simulink model "usv_sys"  (R2023b)
settings: Solver=VariableStepAuto  StartTime=0.0  StopTime=200  RelTol=1e-3
libraries: slpidlib x1
settings Model: Creator=hw  LastModifiedBy=hw

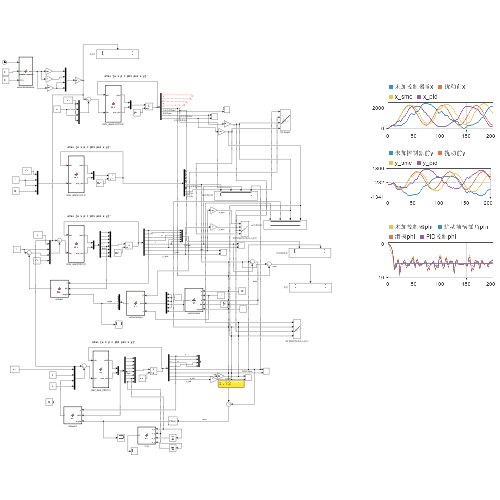
[thumbnail: Simulink's stored preview of the top-level diagram]
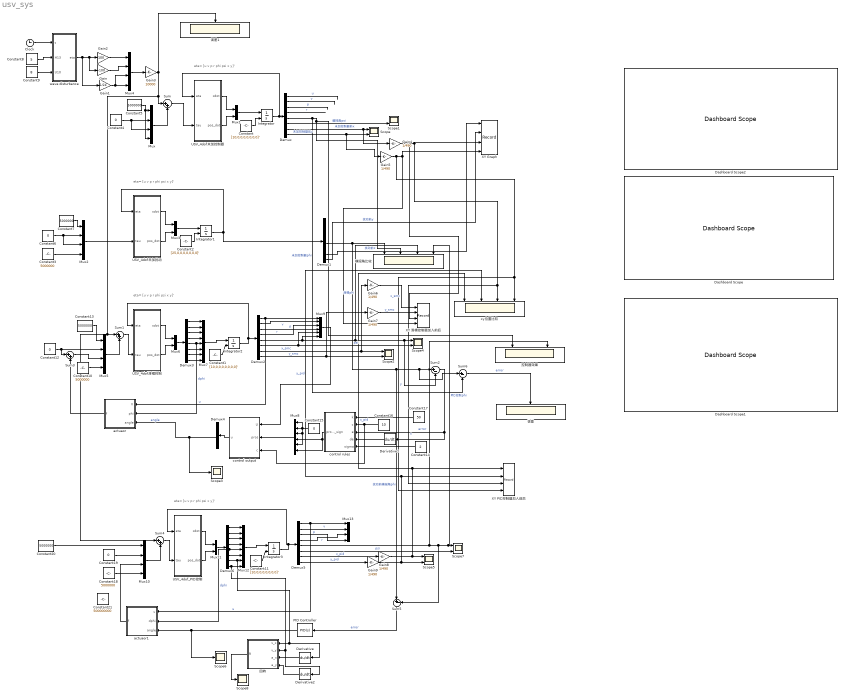
== system usv_sys ==
  note: eta= [u v p r phi psi x y]'
  note: eta= [u v p r phi psi x y]'
  note: eta= [u v p r phi psi x y]'
  note: eta= [u v p r phi psi x y]'
  Clock : Clock
  Constant : Constant  Value=[10,0,0,0,0,0,0,0]'  VectorParams1D=off
  Constant1 : Constant  Value=[10,0,0,0,0,0,0,0]'  VectorParams1D=off
  Constant{3,5,7,10,13,18,20} (7 alike) : Constant  Value=5000000
  Constant11 : Constant  Value=[10,0,0,0,0,0,0,0]'  VectorParams1D=off
  Constant{4,6,12,15,19} (5 alike) : Constant  Value=0
  Constant14 : Constant  Value=2
  Constant16 : Constant  Value=10
  Constant17 : Constant  Value=50
  Constant2 : Constant  Value=[25,0,0,0,0,0,0,0]'  VectorParams1D=off
  Constant21 : Constant  Value=500000000
  Constant8 : Constant  Value=5
  Constant9 : Constant  Value=8
  Dashboard Scope : DashboardScope
  Dashboard Scope1 : DashboardScope
  Dashboard Scope2 : DashboardScope
  Demux{,1..3,5..6} (6 alike) : Demux  Outputs=8
  Demux4 : Demux  Outputs=6
  Derivative : Derivative
  Derivative1 : Derivative
  Derivative2 : Derivative
  Gain : Gain  Gain=-100
  Gain1 : Gain  Gain=1/24
  Gain2 : Gain  Gain=100
  Gain3 : Gain  Gain=10000
  Gain{4..9} (6 alike) : Gain  Gain=1/490
  Integrator{,1..3} (4 alike) : Integrator  InitialConditionSource=external
  Mux{,2,4..5,10,13} (6 alike) : Mux
  Mux{1,3,6,11} (4 alike) : Mux  Inputs=2
  Mux12 : Mux  Inputs=8
  Mux7 : Mux  Inputs=8
  Mux8 : Mux  Inputs=6
  Mux9 : Mux  Inputs=6
  PID Controller : slpidlib/PID Controller  Controller=PID  Form=Parallel  TimeDomain=Continuous-time  UseExternalTs=off  SampleTime=-1  IntegratorMethod=Forward Euler  FilterMethod=Forward Euler  ControllerParametersSource=internal  P=5  I=0.01  UseKiTs=off  D=2  N=100  UseFilter=on  TunerSelectOption=Transfer Function Based (PID Tuner App)  InitialConditionSource=internal  InitialConditionForIntegrator=0  InitialConditionForFilter=0  DifferentiatorICPrevScaledInput=0  ExternalReset=none  TrackingMode=off  Kt=1  LimitOutput=off  SatLimitsSource=internal  UpperSaturationLimit=inf  LowerSaturationLimit=-inf  LinearizeAsGain=on  AntiWindupMode=none  Kb=1  LimitIntegrator=off  UpperIntegratorSaturationLimit=inf  LowerIntegratorSaturationLimit=-inf  POutMin=[]  POutMax=[]  IOutMin=[]  IOutMax=[]  DOutMin=[]  DOutMax=[]  NOutMin=[]  NOutMax=[]  SumOutMin=[-15]  SumOutMax=[15]  SaturationOutMin=[]  SaturationOutMax=[]  PParamMin=[]  PParamMax=[]  IParamMin=[]  IParamMax=[]  DParamMin=[]  DParamMax=[]  NParamMin=[]  NParamMax=[]  KbParamMin=[]  KbParamMax=[]  KtParamMin=[]  KtParamMax=[]  KbOutMin=[]  KbOutMax=[]  KtOutMin=[]  KtOutMax=[]  IntegratorOutMin=[]  IntegratorOutMax=[]  FilterOutMin=[]  FilterOutMax=[]  SumI1OutMin=[]  SumI1OutMax=[]  SumI2OutMin=[]  SumI2OutMax=[]  SumI3OutMin=[]  SumI3OutMax=[]  SumI4OutMin=[]  SumI4OutMax=[]  SumDOutMin=[]  SumDOutMax=[]  DifferentiatorOutMin=[]  DifferentiatorOutMax=[]  FilterDiffOutCoefMin=[]  FilterDiffOutCoefMax=[]  ReciprocalOutMin=[]  ReciprocalOutMax=[]  SumDenOutMin=[]  SumDenOutMax=[]  SumNumOutMin=[]  SumNumOutMax=[]  DivideOutMin=[]  DivideOutMax=[]  UdiffTsProdOutMin=[]  UdiffTsProdOutMax=[]  NTsProdOutMin=[]  NTsProdOutMax=[]  UintegralTsProdOutMin=[]  UintegralTsProdOutMax=[]  UngainTsProdOutMin=[]  UngainTsProdOutMax=[]  ClampingZeroOutDataTypeStr=Inherit: Inherit via back propagation  ClampingZeroOutMin=[]  ClampingZeroOutMax=[]  FilterDenConstantOutDataTypeStr=Inherit: Inherit via back propagation  FilterDenConstantOutMin=[]  FilterDenConstantOutMax=[]  PCopyOutDataTypeStr=Inherit: Inherit via back propagation  PCopyOutMin=[]  PCopyOutMax=[]  NCopyOutDataTypeStr=Inherit: Inherit via back propagation  NCopyOutMin=[]  NCopyOutMax=[]  IntegratorContinuousStateAttributes=''  IntegratorStateMustResolveToSignalObject=off  IntegratorRTWStateStorageClass=Auto  FilterContinuousStateAttributes=''  FilterStateMustResolveToSignalObject=off  FilterRTWStateStorageClass=Auto  ParallelPVariant=InternalParameters  IdealPVariant=Disabled  IVariant=InternalParameters  DVariant=InternalParameters  IntegratorVariant=Continuous  SatVariant=Disabled  AWVariant=Passthrough  PCopyVariant=Disabled  TRVariant=Disabled  FdbkBlocksVariant=Forward  IdealPFdbkVariant=Disabled  SatFdbkVariant=Disabled  DerivativeFilterVariant=ContFilter  NVariant=InternalParameters  NCopyVariant=Disabled  FilterICVariant=InternalICsFilter  IntegratorICVariant=InternalICs  ExternalResetVariant=Disabled  TRSumVariant=Passthrough  SumFdbkVariant=Disabled  SumVariant=Sum_PID  TsampFilterVariant=InternalTs  TsampNgainVariant=Passthrough  TsampIntegralVariant=Disabled_SignalSpec  ExternalSaturationOutDataTypeStr=Inherit: Same as second input
  Scope{,1..2,4..5,7} (6 alike) : Scope  NumInputPorts=2
  Scope3 : Scope
  Scope6 : Scope
  Scope8 : Scope
  Sum{,1,3..4} (4 alike) : Sum  Inputs=|++
  Sum2 : Sum  Inputs=|+-
  Sum5 : Sum  Inputs=|+-
  Sum6 : Sum  Inputs=|+-
  USV_4dof_PID控制 : MATLAB Function  TreatAsAtomicUnit=on
  USV_4dof未加扰动 : MATLAB Function  TreatAsAtomicUnit=on
  USV_4dof未加控制器 : MATLAB Function  TreatAsAtomicUnit=on
  USV_4dof滑模控制 : MATLAB Function  TreatAsAtomicUnit=on
  XY Graph : Record  RecordToFile=on  FileSettingsInternal="{\"entries\":[{\"content\":{\"excelSettings\":{\"content\":{},\"type\":\"Streamout.ExcelSettings\"}},\"type\":\"Streamout.FileSettingStorage\",\"uuid\":\"\"}],\"packageUris\":[\"http:\\/\\/schema.mathworks.com\\/mf0\\/streamout_blocks\\/R2020a\"],\"version\":\"1.0\"}"  Layout=[1 1]  SignalsInternal="{\"entries\":[{\"content\":{\"signals\":[{\"content\":{\"blockPath\":[],\"dimensions\":[1,1],\"domain\":\"\",\"lineColor\":\"#ff6929\",\"plots\":[1],\"port\":1,\"sid\":[\"\"],\"signalID\":6587,\"signalName\":\"扰动前x\"},\"type\":\"RecordBlkView.Signal\",\"uuid\":\"\"},{\"content\":{\"blockPath\":[],\"dimensions\":[1,1],\"domain\":\"\",\"lineColor\":\"#b746ff\",\"plots\":[1],\"port\":2,\"sid\":[\"\"],\"signalID\":6591,\"signalName\":\"扰动前y\"},\"type\":\"RecordBlkView.Signal\",\"uuid\":\"\"},{\"content\":{\"blockPath\":[],\"dimensions\":[1,1],\"domain\":\"\",\"lineColor\":\"#edb120\",\"port\":3,\"sid\":[\"\"],\"signalID\":6595,\"signalName\":\"x\"},\"type\":\"RecordBlkView.Signal\",\"uuid\":\"\"},{\"content\":{\"blockPath\":[],\"dimensions\":[1,1],\"domain\":\"\",\"lineColor\":\"#7e2f8e\",\"port\":4,\"sid\":[\"\"],\"signalID\":6599,\"signalName\":\"y\"},\"type\":\"RecordBlkView.Signal\",\"uuid\":\"\"}]},\"type\":\"RecordBlkView.InputSignals\",\"uuid\":\"\"}],\"packageUris\":[\"http:\\/\\/schema.mathworks.com\\/mf0\\/streamout_blocks\\/R2020a\"],\"version\":\"1.0\"}"  VisualizationBindings="{\"xyplotplugin\":{\"info\":[{\"series\":[{\"bindingParametersList\":[{\"parameter\":\"X-Axis\",\"signalID\":6587,\"signalName\":\"扰动前x\"},{\"parameter\":\"Y-Axis\",\"signalID\":6591,\"signalName\":\"扰动前y\"}],\"seriesID\":62716}],\"subplotID\":1}]}}"  CompatibilityTag=XY
  XY PID控制器加入前后 : Record  FileSettingsInternal="{\"entries\":[{\"content\":{\"excelSettings\":{\"content\":{},\"type\":\"Streamout.ExcelSettings\"}},\"type\":\"Streamout.FileSettingStorage\",\"uuid\":\"\"}],\"packageUris\":[\"http:\\/\\/schema.mathworks.com\\/mf0\\/streamout_blocks\\/R2020a\"],\"version\":\"1.0\"}"  Layout=[1 1]  SignalsInternal="{\"entries\":[{\"content\":{\"signals\":[{\"content\":{\"blockPath\":[],\"dimensions\":[1,1],\"domain\":\"\",\"lineColor\":\"#77ac30\",\"port\":1,\"sid\":[\"\"],\"signalID\":6603,\"signalName\":\"x_pid\"},\"type\":\"RecordBlkView.Signal\",\"uuid\":\"\"},{\"content\":{\"blockPath\":[],\"dimensions\":[1,1],\"domain\":\"\",\"lineColor\":\"#4dbeee\",\"port\":2,\"sid\":[\"\"],\"signalID\":6607,\"signalName\":\"y_pid\"},\"type\":\"RecordBlkView.Signal\",\"uuid\":\"\"},{\"content\":{\"blockPath\":[],\"dimensions\":[1,1],\"domain\":\"\",\"lineColor\":\"#a2142f\",\"port\":3,\"sid\":[\"\"],\"signalID\":6611,\"signalName\":\"x\"},\"type\":\"RecordBlkView.Signal\",\"uuid\":\"\"},{\"content\":{\"blockPath\":[],\"dimensions\":[1,1],\"domain\":\"\",\"lineColor\":\"#139fff\",\"port\":4,\"sid\":[\"\"],\"signalID\":6615,\"signalName\":\"y\"},\"type\":\"RecordBlkView.Signal\",\"uuid\":\"\"}]},\"type\":\"RecordBlkView.InputSignals\",\"uuid\":\"\"}],\"packageUris\":[\"http:\\/\\/schema.mathworks.com\\/mf0\\/streamout_blocks\\/R2020a\"],\"version\":\"1.0\"}"  VisualizationBindings="{\"xyplotplugin\":{\"info\":[{\"series\":[],\"subplotID\":1}]}}"  CompatibilityTag=XY
  XY 滑模控制器加入前后 : Record  FileSettingsInternal="{\"entries\":[{\"content\":{\"excelSettings\":{\"content\":{},\"type\":\"Streamout.ExcelSettings\"}},\"type\":\"Streamout.FileSettingStorage\",\"uuid\":\"\"}],\"packageUris\":[\"http:\\/\\/schema.mathworks.com\\/mf0\\/streamout_blocks\\/R2020a\"],\"version\":\"1.0\"}"  Layout=[1 1]  SignalsInternal="{\"entries\":[{\"content\":{\"signals\":[{\"content\":{\"blockPath\":[],\"dimensions\":[1,1],\"domain\":\"\",\"lineColor\":\"#4dbeee\",\"port\":1,\"sid\":[\"\"],\"signalID\":6619,\"signalName\":\"x_smc\"},\"type\":\"RecordBlkView.Signal\",\"uuid\":\"\"},{\"content\":{\"blockPath\":[],\"dimensions\":[1,1],\"domain\":\"\",\"lineColor\":\"#a2142f\",\"port\":2,\"sid\":[\"\"],\"signalID\":6623,\"signalName\":\"y_smc\"},\"type\":\"RecordBlkView.Signal\",\"uuid\":\"\"},{\"content\":{\"blockPath\":[],\"dimensions\":[1,1],\"domain\":\"\",\"lineColor\":\"#139fff\",\"port\":3,\"sid\":[\"\"],\"signalID\":6627,\"signalName\":\"x\"},\"type\":\"RecordBlkView.Signal\",\"uuid\":\"\"},{\"content\":{\"blockPath\":[],\"dimensions\":[1,1],\"domain\":\"\",\"lineColor\":\"#ff6929\",\"port\":4,\"sid\":[\"\"],\"signalID\":6631,\"signalName\":\"y\"},\"type\":\"RecordBlkView.Signal\",\"uuid\":\"\"}]},\"type\":\"RecordBlkView.InputSignals\",\"uuid\":\"\"}],\"packageUris\":[\"http:\\/\\/schema.mathworks.com\\/mf0\\/streamout_blocks\\/R2020a\"],\"version\":\"1.0\"}"  VisualizationBindings="{\"xyplotplugin\":{\"info\":[{\"series\":[],\"subplotID\":1}]}}"  CompatibilityTag=XY
  actuaor : MATLAB Function  TreatAsAtomicUnit=on
  actuaor1 : MATLAB Function  TreatAsAtomicUnit=on
  control output : MATLAB Function  TreatAsAtomicUnit=on
  control rules : MATLAB Function  TreatAsAtomicUnit=on
  wave disturbance : MATLAB Function  TreatAsAtomicUnit=on
  xy位置比较 : Scope  NumInputPorts=4
  回转 : MATLAB Function  TreatAsAtomicUnit=on
  控制器效果 : Scope  NumInputPorts=2
  横摇角比较 : Scope  NumInputPorts=4
  误差 : Scope
  误差1 : Scope
  wires:
  Constant/1 -> Integrator/2
  Constant4/1 -> Mux/3, Mux/2
  USV_4dof未加控制器/1(xdot) -> Mux1/1
  Demux/7 -> Gain4/1, Scope/1  "未加控制器前x"
  Demux/8 -> Gain5/1, Scope/2  "未加控制器前y"
  USV_4dof未加控制器/2(pos_dot) -> Mux1/2
  Constant5/1 -> Mux/4, Mux/1
  Integrator/1 -> USV_4dof未加控制器/1(eta), Demux/1
  Mux/1 -> Sum/2
  Mux1/1 -> Integrator/1
  Demux/1 -> ?  "u"
  Demux/2 -> ?  "v"
  Demux/3 -> ?  "p"
  Demux/4 -> ?  "r"
  Demux/6 -> Scope1/2  "艏摇角psi"
  Mux2/1 -> USV_4dof未加扰动/2(tau)
  USV_4dof未加扰动/2(pos_dot) -> Mux3/2
  Constant3/1 -> Mux2/4
  Constant7/1 -> Mux2/1
  USV_4dof未加扰动/1(xdot) -> Mux3/1
  Constant2/1 -> Integrator1/2
  Integrator1/1 -> USV_4dof未加扰动/1(eta), Demux1/1
  Constant6/1 -> Mux2/3, Mux2/2
  Mux3/1 -> Integrator1/1
  Constant9/1 -> wave disturbance/3(U10)
  Mux4/1 -> Gain3/1
  Gain1/1 -> Mux4/3, Mux4/4
  Clock/1 -> wave disturbance/1(t)
  Gain2/1 -> Mux4/1
  Constant8/1 -> wave disturbance/2(H13)
  wave disturbance/1(eta) -> Gain1/1, Gain/1, Gain2/1
  Sum/1 -> USV_4dof未加控制器/2(tau)
  Gain4/1 -> XY 滑模控制器加入前后/3, XY PID控制器加入前后/3, xy位置比较/3, XY Graph/3  "x"
  Gain5/1 -> XY PID控制器加入前后/4, xy位置比较/4, XY 滑模控制器加入前后/4, XY Graph/4  "y"
  Demux/5 -> Sum6/2, 控制器效果/1, 横摇角比较/2  "未加控制器phi"
  Demux1/5 -> Sum5/1, Sum6/1, Sum2/1, 横摇角比较/1  "扰动前横摇角phi"
  Demux2/6 -> Mux9/5, Scope4/2  "psi"
  Demux2/7 -> Scope2/1, Gain6/1  "x_smc"
  USV_4dof滑模控制/2(pos_dot) -> Mux6/2
  Demux2/4 -> Mux9/3  "r"
  Demux4/4 -> Scope3/1, actuaor/3(angle)  "angle"
  Constant13/1 -> Mux5/1
  Derivative1/1 -> control rules/4(de)
  Mux7/1 -> Integrator2/1
  Mux8/1 -> control output/2(pros)
  Demux3/7 -> Mux7/7
  Mux9/1 -> control output/1(U)
  Demux3/3 -> Mux7/3
  Demux2/2 -> Mux9/2  "v"
  Demux3/5 -> actuaor/2(phi), Mux7/5  "dphi"
  Constant17/1 -> control rules/1(k)
  Constant12/1 -> Sum3/1, Mux5/2
  Constant14/1 -> control rules/5(sigma)
  Demux2/1 -> actuaor/1(V), Mux9/1  "u"
  control rules/1(prox1_sign) -> Mux8/6, Mux8/4
  Sum2/1 -> Derivative1/1, control rules/3(e)  "error"
  Demux2/8 -> Gain7/1, Scope2/2  "y_smc"
  Constant1/1 -> Integrator2/2
  Sum3/1 -> Mux5/3
  Demux2/5 -> Mux9/6, Sum2/2, Scope4/1, 横摇角比较/3  "滑模phi"
  Demux3/6 -> Mux7/6
  Demux3/4 -> Mux7/4
  Demux2/3 -> Mux9/4  "p"
  Demux3/1 -> Mux7/1
  Constant15/1 -> Mux8/1, Mux8/5, Mux8/3, Mux8/2
  Demux3/2 -> Mux7/2
  Mux6/1 -> Demux3/1
  Constant16/1 -> control output/3(c), control rules/2(c)
  Constant10/1 -> Mux5/4
  Integrator2/1 -> USV_4dof滑模控制/1(eta), Demux2/1
  Demux3/8 -> Mux7/8
  actuaor/1(f) -> Sum3/2
  USV_4dof滑模控制/1(xdot) -> Mux6/1
  Mux5/1 -> Sum1/2
  Sum1/1 -> USV_4dof滑模控制/2(tau)
  control output/1(u) -> Demux4/1
  actuaor1/1(f) -> Mux10/3
  Gain3/1 -> Sum4/1, Sum1/1, Sum/1, 误差1/1
  回转/1(R) -> Scope8/1
  Integrator3/1 -> USV_4dof_PID控制/1(eta), Demux5/1
  Constant11/1 -> Integrator3/2
  USV_4dof_PID控制/2(pos_dot) -> Mux11/2
  Demux6/7 -> 回转/1(v_x), Derivative/1, Mux12/7
  Demux6/5 -> Mux12/5, actuaor1/2(dphi)  "dphi"
  Mux11/1 -> Demux6/1
  Demux6/2 -> Mux12/2
  Mux12/1 -> Integrator3/1
  PID Controller/1 -> Scope6/1, actuaor1/3(angle)
  Demux6/4 -> Mux12/4
  Demux5/5 -> 控制器效果/2, 横摇角比较/4, Scope7/1, Sum5/2  "PID控制phi"
  Constant18/1 -> Mux10/4
  Demux6/3 -> Mux12/3
  Demux5/8 -> Gain9/1  "y_pid"
  Demux5/1 -> Mux13/1, actuaor1/1(v)  "u"
  Demux5/4 -> Mux13/3  "r"
  Demux5/6 -> Scope7/2  "psi"
  Demux6/8 -> Derivative2/1, 回转/2(v_y), Mux12/8
  Demux5/2 -> Mux13/2  "v"
  Demux5/7 -> Gain8/1  "x_pid"
  Mux10/1 -> Sum4/2
  Constant20/1 -> Mux10/1
  Sum5/1 -> PID Controller/1  "error"
  Demux6/6 -> Mux12/6
  Derivative/1 -> 回转/3(a_x)
  Sum4/1 -> USV_4dof_PID控制/2(tau)
  USV_4dof_PID控制/1(xdot) -> Mux11/1
  Demux6/1 -> Mux12/1
  Constant19/1 -> Mux10/2
  Demux5/3 -> Mux13/4  "p"
  Derivative2/1 -> 回转/4(a_y)
  Gain/1 -> Mux4/2
  Gain6/1 -> XY 滑模控制器加入前后/1  "x_smc"
  Gain7/1 -> XY 滑模控制器加入前后/2  "y_smc"
  Gain8/1 -> XY PID控制器加入前后/1, xy位置比较/1, Scope5/1  "x_pid"
  Gain9/1 -> XY PID控制器加入前后/2, xy位置比较/2, Scope5/2  "y_pid"
  Sum6/1 -> 误差/1  "error"
  Demux1/7 -> XY Graph/1  "扰动前x"
  Demux1/8 -> XY Graph/2  "扰动前y"

== matlab function usv_sys/USV_4dof未加控制器 ==
  data: eta input size=8*1; xdot output size=6*1; tau input; pos_dot output size=2*1
function [xdot,pos_dot] = usv(eta, tau)

% 线性化船舶模型
% Inputs:
% eta= [u v p r phi psi x y]'
% xdot= [du dv dp dr dphi dpsi]'
% pos_dot=[dx dy]'
% tau = [Xe Ye Ke Ne]' 
%

% where
% u     = surge velocity          (m/s)
% v     = sway velocity           (m/s)
% p     = roll velocity           (rad/s)
% r     = yaw velocity            (rad/s)
% phi   = roll angle              (rad)
% psi   = yaw angle               (rad)
%
% Xe is the surge external force (e.g. rudder and fin forces)
% Ye is the sway external force  
% Ke is the sway external force  
% Ne is the sway external force   

% Vessel Data
rho_water     =	1014.0;	        %	water density	[kg/m^3]	
rho_air		=	1.225	;	    %	air density		[kg/m^3]	
g				=	9.81;	        %	gravity constant	[m/s^2]	
deg2rad 		=	pi/180;	        %	degrees to radians	
rad2deg 		=	180/pi;	        %	rad to degrees		
ms2kt			=	3600/1852;	    % 	m/s to kt 			
kt2ms 		=	1852/3600;	    %	kt to m/s			
RPM2rads		=	2*pi/60;	    %	RPM to rad/s		
rads2RPM		=   60/(2*pi);	    %	rad/s to RPM		
HP2W			=	745.700;	    %	HP to Watt			


Lpp    =  51.5 ;                  % Length between perpendiculars垂直间长 [m]
B      =  8.6  ;                  % Beam over all 船宽 [m]
D	   =  2.3  ;                  % Draught吃水深度 [m]     

%Load condition (Modified by T.Perez)
disp   =  350.0;                   % Displacement 排水量 [m^3]
m      =  disp*rho_water;          % Mass [Kg]
Izz    =  47.934*10^6 ;            % Yaw Inertia偏航转动惯量
Ixx    =  2.3763*10^6 ;            % Roll Inertia横滚转动惯量
U_nom  =  8.0   ;	               % Speed nominal [m/sec]速度 (app 15kts) 
KM		=  4.47;	             %  [m] Transverse metacentre above keel 横倾复原力臂
KB		=  1.53;	             %  [m] Transverse centre of bouancy 浮心高度
gm 		=  1.1;	                 %  [m]	Transverse Metacenter 
bm 		=  KM - KB;
LCG       = 20.41 ;                % [m]	Longitudinal CG (from AP considered at the rudder stock)
VCG       = 3.36  ;                % [m]	Vertical  CG  above baseline
xG        = -3.38  ;               % coordinate of CG from the body fixed frame adopted for the PMM test  
zG  	    = -(VCG-D);          % coordinate of CG from the body fixed frame adopted for the PMM test  
m_xg	    = m * xG;
m_zg	    = m * zG;
Dp        = 1.6 ;                   % Propeller diameter [m]


% Data for surge equation 纵向（均为线性流体动力导数）
Xudot  	= -17400.0 ;  %-mx
Xuau     	= -1.96e+003 ;
Xvr    	=  0.33 * m ;
   
% Hydrodynamic coefficients in sway equation横向
Yvdot = -393000 ;  %-my
Ypdot = -296000 ; 
Yrdot = -1400000 ; %附加质量静距
Yauv  = -11800 ; 
Yur   =  131000 ; 
Yvav  = -3700 ; 
Yrar   =  0 ;
Yvar  = -794000 ; 
Yrav  = -182000 ; 
Ybauv =  10800 ; % Y_{\phi |v u|}
Ybaur =  251000 ; 
Ybuu  = -74 ; 


% Hydrodynamic coefficients in roll equation横摇水动力系数
Kvdot =  296000 ;
Kpdot = -774000 ;  %-Jxx
Krdot =  0 ;
Kauv  =  9260 ;
Kur   = -102000 ;
Kvav  =  29300 ;
Krar  =  0 ;
Kvar  =  621000 ;
Krav  =  142000 ;
Kbauv =  -8400 ;
Kbaur =  -196000 ;
Kbuu  =  -1180 ;
Kaup  =  -15500 ;
Kpap  =  -416000 ;
Kp    =  -500000 ;
Kb    =  0.776*m*g;
Kbbb  =  -0.325*m*g ;

% Hydrodynamic coefficients in yaw equation偏航水动力系数
Nvdot =  538000 ;   %-
Npdot =  0 ;
Nrdot = -38.7e6;    %jzz
Nauv  = -92000 ;
Naur  = -4710000 ;
Nvav  =  0 ;
Nrar  = -202000000 ;
Nvar  =  0 ;
Nrav  = -15600000 ;
Nbauv = -214000 ;
Nbuar = -4980000 ;
Nbuau = -8000 ;
%%%%%%%%%%%%%%%%%%%%%%%%%%%%%%%%%%%%%%%%%%%%%%%%%%%%%%%%%%%%%%%%%%%%%%%%%%%

% 定义输入
u   = eta(1);
v   = eta(2);
p  	= eta(3);   	
r  	= eta(4); 
b  	= eta(5); %phi roll 		
psi = eta(6);
x  	= eta(7);   	
y  	= eta(8); 
% 外部力与力矩
Xe  = tau(1);
Ye  = tau(2);
Ke  = tau(3);
Ne  = tau(4);

% Auxiliary variables辅助变量
au = abs(u);
av = abs(v); 
ar = abs(r); 
ap = abs(p); 
ab = abs(b);
L2 = Lpp^2; %参考面积？

% Total Mass Matrix 刚体质量矩阵
% x= [u v p r phi psi ]'
M =[ (m-Xudot)  0   0   0   0   0;
   0 (m-Yvdot) -(m*zG+Ypdot) (m*xG-Yrdot) 0 0;
   0 -(m*zG+Kvdot) (Ixx-Kpdot) -Krdot 0 0;
   0 (m*xG-Nvdot) -Npdot (Izz-Nrdot) 0 0;
   0 0 0 0 1 0; 
   0 0 0 0 0 1] ;
%转换矩阵
J=[cos(psi),-cos(b)*sin(psi);sin(psi),cos(b)*cos(psi)];
X=[u,v]';   
% Hydrodynamic forces without added mass terms(considered in the M matrix)
% 不考虑附加质量的水动力作用力 粘性流动动力（贵岛模型）
Xh  = Xuau*u*au+Xvr*v*r;

Yh = Yauv*au*v +  Yur*u*r + Yvav*v*av + Yvar*v*ar + Yrav*r*av + Ybauv*b*abs(u*v) + Ybaur*b*abs(u*r) + Ybuu*b*u^2;

Kh = Kauv*au*v +Kur*u*r + Kvav*v*av + Kvar*v*ar + Krav*r*av + Kbauv*b*abs(u*v) + Kbaur*b*abs(u*r) + Kbuu*b*u^2 +Kaup*au*p + Kpap*p*ap +Kp*p +Kbbb*b^3-(rho_water*g*gm*disp)*b;

Nh =Nauv*au*v + Naur*au*r +Nrar*r*ar + Nrav*r*av+Nbauv*b*abs(u*b) + Nbuar*b*u*ar + Nbuau*b*u*au;
 
% Rigid-body centripetal accelerations刚体运动产生的离心加速度影响
Xc =  m*(r*v+xG*r^2-zG*p*r);  
Yc = - m*u*r;
Kc =   m*zG*u*r;
Nc = - m*xG*u*r;

% Total forces
F1 = Xh+Xc+Xe;
F2 = Yh+Yc+Ye;
F4 = Kh+Kc+Ke;
F6 = Nh+Nc+Ne;

%运动学及动力学方程
pos_dot=J*X;
xdot = M\[F1; F2; F4; F6; p; r*cos(b)];

end

== matlab function usv_sys/USV_4dof未加扰动 ==
  data: eta input size=8*1; xdot output size=6*1; tau input; pos_dot output size=2*1
function [xdot,pos_dot] = usv(eta, tau)

% 线性化船舶模型
% Inputs:
% eta= [u v p r phi psi x y]'
% xdot= [du dv dp dr dphi dpsi]'
% pos_dot=[dx dy]'
% tau = [Xe Ye Ke Ne]' 
%

% where
% u     = surge velocity          (m/s)
% v     = sway velocity           (m/s)
% p     = roll velocity           (rad/s)
% r     = yaw velocity            (rad/s)
% phi   = roll angle              (rad)
% psi   = yaw angle               (rad)
%
% Xe is the surge external force (e.g. rudder and fin forces)
% Ye is the sway external force  
% Ke is the sway external force  
% Ne is the sway external force   

% Vessel Data
rho_water     =	1014.0;	        %	water density	[kg/m^3]	
rho_air		=	1.225	;	    %	air density		[kg/m^3]	
g				=	9.81;	        %	gravity constant	[m/s^2]	
deg2rad 		=	pi/180;	        %	degrees to radians	
rad2deg 		=	180/pi;	        %	rad to degrees		
ms2kt			=	3600/1852;	    % 	m/s to kt 			
kt2ms 		=	1852/3600;	    %	kt to m/s			
RPM2rads		=	2*pi/60;	    %	RPM to rad/s		
rads2RPM		=   60/(2*pi);	    %	rad/s to RPM		
HP2W			=	745.700;	    %	HP to Watt			


Lpp    =  51.5 ;                  % Length between perpendiculars垂直间长 [m]
B      =  8.6  ;                  % Beam over all 船宽 [m]
D	   =  2.3  ;                  % Draught吃水深度 [m]     

%Load condition (Modified by T.Perez)
disp   =  350.0;                   % Displacement 排水量 [m^3]
m      =  disp*rho_water;          % Mass [Kg]
Izz    =  47.934*10^6 ;            % Yaw Inertia偏航转动惯量
Ixx    =  2.3763*10^6 ;            % Roll Inertia横滚转动惯量
U_nom  =  8.0   ;	               % Speed nominal [m/sec]速度 (app 15kts) 
KM		=  4.47;	             %  [m] Transverse metacentre above keel 横倾复原力臂
KB		=  1.53;	             %  [m] Transverse centre of bouancy 浮心高度
gm 		=  1.1;	                 %  [m]	Transverse Metacenter 
bm 		=  KM - KB;
LCG       = 20.41 ;                % [m]	Longitudinal CG (from AP considered at the rudder stock)
VCG       = 3.36  ;                % [m]	Vertical  CG  above baseline
xG        = -3.38  ;               % coordinate of CG from the body fixed frame adopted for the PMM test  
zG  	    = -(VCG-D);          % coordinate of CG from the body fixed frame adopted for the PMM test  
m_xg	    = m * xG;
m_zg	    = m * zG;
Dp        = 1.6 ;                   % Propeller diameter [m]


% Data for surge equation 纵向（均为线性流体动力导数）
Xudot  	= -17400.0 ;  %-mx
Xuau     	= -1.96e+003 ;
Xvr    	=  0.33 * m ;
   
% Hydrodynamic coefficients in sway equation横向
Yvdot = -393000 ;  %-my
Ypdot = -296000 ; 
Yrdot = -1400000 ; %附加质量静距
Yauv  = -11800 ; 
Yur   =  131000 ; 
Yvav  = -3700 ; 
Yrar   =  0 ;
Yvar  = -794000 ; 
Yrav  = -182000 ; 
Ybauv =  10800 ; % Y_{\phi |v u|}
Ybaur =  251000 ; 
Ybuu  = -74 ; 


% Hydrodynamic coefficients in roll equation横摇水动力系数
Kvdot =  296000 ;
Kpdot = -774000 ;  %-Jxx
Krdot =  0 ;
Kauv  =  9260 ;
Kur   = -102000 ;
Kvav  =  29300 ;
Krar  =  0 ;
Kvar  =  621000 ;
Krav  =  142000 ;
Kbauv =  -8400 ;
Kbaur =  -196000 ;
Kbuu  =  -1180 ;
Kaup  =  -15500 ;
Kpap  =  -416000 ;
Kp    =  -500000 ;
Kb    =  0.776*m*g;
Kbbb  =  -0.325*m*g ;

% Hydrodynamic coefficients in yaw equation偏航水动力系数
Nvdot =  538000 ;   %-
Npdot =  0 ;
Nrdot = -38.7e6;    %jzz
Nauv  = -92000 ;
Naur  = -4710000 ;
Nvav  =  0 ;
Nrar  = -202000000 ;
Nvar  =  0 ;
Nrav  = -15600000 ;
Nbauv = -214000 ;
Nbuar = -4980000 ;
Nbuau = -8000 ;
%%%%%%%%%%%%%%%%%%%%%%%%%%%%%%%%%%%%%%%%%%%%%%%%%%%%%%%%%%%%%%%%%%%%%%%%%%%

% 定义输入
u   = eta(1);
v   = eta(2);
p  	= eta(3);   	
r  	= eta(4); 
b  	= eta(5); %phi roll 		
psi = eta(6);
x  	= eta(7);   	
y  	= eta(8); 
% 外部力与力矩
Xe  = tau(1);
Ye  = tau(2);
Ke  = tau(3);
Ne  = tau(4);

% Auxiliary variables辅助变量
au = abs(u);
av = abs(v); 
ar = abs(r); 
ap = abs(p); 
ab = abs(b);
L2 = Lpp^2; %参考面积？

% Total Mass Matrix 刚体质量矩阵
% x= [u v p r phi psi ]'
M =[ (m-Xudot)  0   0   0   0   0;
   0 (m-Yvdot) -(m*zG+Ypdot) (m*xG-Yrdot) 0 0;
   0 -(m*zG+Kvdot) (Ixx-Kpdot) -Krdot 0 0;
   0 (m*xG-Nvdot) -Npdot (Izz-Nrdot) 0 0;
   0 0 0 0 1 0; 
   0 0 0 0 0 1] ;
%转换矩阵
J=[cos(psi),-cos(b)*sin(psi);sin(psi),cos(b)*cos(psi)];
X=[u,v]';   
% Hydrodynamic forces without added mass terms(considered in the M matrix)
% 不考虑附加质量的水动力作用力 粘性流动动力（贵岛模型）
Xh  = Xuau*u*au+Xvr*v*r;

Yh = Yauv*au*v +  Yur*u*r + Yvav*v*av + Yvar*v*ar + Yrav*r*av + Ybauv*b*abs(u*v) + Ybaur*b*abs(u*r) + Ybuu*b*u^2;

Kh = Kauv*au*v +Kur*u*r + Kvav*v*av + Kvar*v*ar + Krav*r*av + Kbauv*b*abs(u*v) + Kbaur*b*abs(u*r) + Kbuu*b*u^2 +Kaup*au*p + Kpap*p*ap +Kp*p +Kbbb*b^3-(rho_water*g*gm*disp)*b;

Nh =Nauv*au*v + Naur*au*r +Nrar*r*ar + Nrav*r*av+Nbauv*b*abs(u*b) + Nbuar*b*u*ar + Nbuau*b*u*au;
 
% Rigid-body centripetal accelerations刚体运动产生的离心加速度影响
Xc =  m*(r*v+xG*r^2-zG*p*r);  
Yc = - m*u*r;
Kc =   m*zG*u*r;
Nc = - m*xG*u*r;

% Total forces
F1 = Xh+Xc+Xe;
F2 = Yh+Yc+Ye;
F4 = Kh+Kc+Ke;
F6 = Nh+Nc+Ne;

%运动学及动力学方程
pos_dot=J*X;
xdot = M\[F1; F2; F4; F6; p; r*cos(b)];

end

== matlab function usv_sys/wave disturbance ==
  settings: updateMethod=DISCRETE
  data: t input; eta output; H13 input; U10 input
function eta = waveGeneration(t, H13, U10)
    % 此函数根据给定的有效波高和风速生成海浪信号
    % 常数定义
    g = 9.81; % 重力加速度, m/s^2
    alpha = 8.11e-3;
    beta = 3.11;
    
    % 风速对应的遭遇频率
    omega_e = 0.84 * (g / U10)^(1/3); % 峰值遭遇频率, rad/s

    % 频率范围和增量
    if H13 <= 2.5
        omegab=0.3;
        omegal =3.0;
        delta_omega = 0.1;
    elseif H13 <= 5.0
        omegab=0.25;
        omegal = 2.4;
        delta_omega = 0.08;
    else 
        omegab=0.1;
        omegal = 1.7;
        delta_omega = 0.06;
    end
    omega = omegab:delta_omega:omegal;

    % 能量密度谱 S(omega)
    S_omega = alpha * g^2 ./ omega.^5 .* exp(-beta ./ (H13^2 * omega.^4));
    % 振幅和相位
    a_omega = sqrt(2 * S_omega * delta_omega);
    phi = rand(1, length(omega)) * 2 * pi;
    % 海浪位移初始化
    eta = zeros(size(t));

    % 构建波形
    for i = 1:length(omega)
        eta = eta + a_omega(i) * cos(omega(i) * t + phi(i));
    end
end

== matlab function usv_sys/USV_4dof滑模控制 ==
  data: eta input size=8*1; xdot output size=6*1; tau input; pos_dot output size=2*1
function [xdot,pos_dot] = usv(eta, tau)

% 线性化船舶模型
% Inputs:
% eta= [u v p r phi psi x y]'
% xdot= [du dv dp dr dphi dpsi]'
% pos_dot=[dx dy]'
% tau = [Xe Ye Ke Ne]' 
%

% where
% u     = surge velocity          (m/s)
% v     = sway velocity           (m/s)
% p     = roll velocity           (rad/s)
% r     = yaw velocity            (rad/s)
% phi   = roll angle              (rad)
% psi   = yaw angle               (rad)
%
% Xe is the surge external force (e.g. rudder and fin forces)
% Ye is the sway external force  
% Ke is the sway external force  
% Ne is the sway external force   

% Vessel Data
rho_water     =	1014.0;	        %	water density	[kg/m^3]	
rho_air		=	1.225	;	    %	air density		[kg/m^3]	
g				=	9.81;	        %	gravity constant	[m/s^2]	
deg2rad 		=	pi/180;	        %	degrees to radians	
rad2deg 		=	180/pi;	        %	rad to degrees		
ms2kt			=	3600/1852;	    % 	m/s to kt 			
kt2ms 		=	1852/3600;	    %	kt to m/s			
RPM2rads		=	2*pi/60;	    %	RPM to rad/s		
rads2RPM		=   60/(2*pi);	    %	rad/s to RPM		
HP2W			=	745.700;	    %	HP to Watt			


Lpp    =  51.5 ;                  % Length between perpendiculars垂直间长 [m]
B      =  8.6  ;                  % Beam over all 船宽 [m]
D	   =  2.3  ;                  % Draught吃水深度 [m]     

%Load condition (Modified by T.Perez)
disp   =  357.0;                   % Displacement 排水量 [m^3]
m      =  disp*rho_water;          % Mass [Kg]
Izz    =  47.934*10^6 ;            % Yaw Inertia偏航转动惯量
Ixx    =  2.3763*10^6 ;            % Roll Inertia横滚转动惯量
U_nom  =  8.0   ;	               % Speed nominal [m/sec]速度 (app 15kts) 
KM		=  4.47;	             %  [m] Transverse metacentre above keel 横倾复原力臂
KB		=  1.53;	             %  [m] Transverse centre of bouancy 浮心高度
gm 		=  1.1;	                 %  [m]	Transverse Metacenter 
bm 		=  KM - KB;
LCG       = 20.41 ;                % [m]	Longitudinal CG (from AP considered at the rudder stock)
VCG       = 3.36  ;                % [m]	Vertical  CG  above baseline
xG        = -3.38  ;               % coordinate of CG from the body fixed frame adopted for the PMM test  
zG  	    = -(VCG-D);          % coordinate of CG from the body fixed frame adopted for the PMM test  
m_xg	    = m * xG;
m_zg	    = m * zG;
Dp        = 1.6 ;                   % Propeller diameter [m]


% Data for surge equation 纵向（均为线性流体动力导数）
Xudot  	= -17400.0 ;  %-mx
Xuau     	= -1.96e+003 ;
Xvr    	=  0.33 * m ;
   
% Hydrodynamic coefficients in sway equation横向
Yvdot = -393000 ;  %-my
Ypdot = -296000 ; 
Yrdot = -1400000 ; %附加质量静距
Yauv  = -11800 ; 
Yur   =  131000 ; 
Yvav  = -3700 ; 
Yrar   =  0 ;
Yvar  = -794000 ; 
Yrav  = -182000 ; 
Ybauv =  10800 ; % Y_{\phi |v u|}
Ybaur =  251000 ; 
Ybuu  = -74 ; 


% Hydrodynamic coefficients in roll equation横摇水动力系数
Kvdot =  296000 ;
Kpdot = -774000 ;  %-Jxx
Krdot =  0 ;
Kauv  =  9260 ;
Kur   = -102000 ;
Kvav  =  29300 ;
Krar  =  0 ;
Kvar  =  621000 ;
Krav  =  142000 ;
Kbauv =  -8400 ;
Kbaur =  -196000 ;
Kbuu  =  -1180 ;
Kaup  =  -15500 ;
Kpap  =  -416000 ;
Kp    =  -500000 ;
Kb    =  0.776*m*g;
Kbbb  =  -0.325*m*g ;

% Hydrodynamic coefficients in yaw equation偏航水动力系数
Nvdot =  538000 ;   %-
Npdot =  0 ;
Nrdot = -38.7e6;    %jzz
Nauv  = -92000 ;
Naur  = -4710000 ;
Nvav  =  0 ;
Nrar  = -202000000 ;
Nvar  =  0 ;
Nrav  = -15600000 ;
Nbauv = -214000 ;
Nbuar = -4980000 ;
Nbuau = -8000 ;
%%%%%%%%%%%%%%%%%%%%%%%%%%%%%%%%%%%%%%%%%%%%%%%%%%%%%%%%%%%%%%%%%%%%%%%%%%%

% 定义输入
u   = eta(1);
v   = eta(2);
p  	= eta(3);   	
r  	= eta(4); 
b  	= eta(5); %phi roll 		
psi = eta(6);
x  	= eta(7);   	
y  	= eta(8); 
% 外部力与力矩
Xe  = tau(1);
Ye  = tau(2);
Ke  = tau(3);
Ne  = tau(4);

% Auxiliary variables辅助变量
au = abs(u);
av = abs(v); 
ar = abs(r); 
ap = abs(p); 
ab = abs(b);
L2 = Lpp^2; %参考面积？

% Total Mass Matrix 刚体质量矩阵
% x= [u v p r phi psi ]'
M =[ (m-Xudot)  0   0   0   0   0;
   0 (m-Yvdot) -(m*zG+Ypdot) (m*xG-Yrdot) 0 0;
   0 -(m*zG+Kvdot) (Ixx-Kpdot) -Krdot 0 0;
   0 (m*xG-Nvdot) -Npdot (Izz-Nrdot) 0 0;
   0 0 0 0 1 0; 
   0 0 0 0 0 1] ;
%转换矩阵
J=[cos(psi),-cos(b)*sin(psi);sin(psi),cos(b)*cos(psi)];
X=[u,v]';   
% Hydrodynamic forces without added mass terms(considered in the M matrix)
% 不考虑附加质量的水动力作用力 粘性流动动力（贵岛模型）
Xh  = Xuau*u*au+Xvr*v*r;

Yh = Yauv*au*v +  Yur*u*r + Yvav*v*av + Yvar*v*ar + Yrav*r*av + Ybauv*b*abs(u*v) + Ybaur*b*abs(u*r) + Ybuu*b*u^2;

Kh = Kauv*au*v +Kur*u*r + Kvav*v*av + Kvar*v*ar + Krav*r*av + Kbauv*b*abs(u*v) + Kbaur*b*abs(u*r) + Kbuu*b*u^2 +Kaup*au*p + Kpap*p*ap +Kp*p +Kbbb*b^3-(rho_water*g*gm*disp)*b;

Nh =Nauv*au*v + Naur*au*r +Nrar*r*ar + Nrav*r*av+Nbauv*b*abs(u*b) + Nbuar*b*u*ar + Nbuau*b*u*au;
 
% Rigid-body centripetal accelerations刚体运动产生的离心加速度影响
Xc =  m*(r*v+xG*r^2-zG*p*r);  
Yc = - m*u*r;
Kc =   m*zG*u*r;
Nc = - m*xG*u*r;

% Total forces
F1 = Xh+Xc+Xe;
F2 = Yh+Yc+Ye;
F4 = Kh+Kc+Ke;
F6 = Nh+Nc+Ne;

%运动学及动力学方程
pos_dot=J*X;
xdot = M\[F1; F2; F4; F6; p; r*cos(b)];

end

== matlab function usv_sys/actuaor ==
  data: V input; phi input; angle input size=1*1; f output size=1*1
function f  = top(V, phi, angle)

d=2;
f=1/2*V^2*1025*10*8.7*(angle+phi*d/V);
end

== matlab function usv_sys/control output ==
  data: U input; u output size=6*1; pros input; c input
function u= fcn(U,pros,c)
A = [-0.0115, 0.0692, -0.0054, 0,0,0 ;
     0, -0.0251, -3.4711, -0.1053, 0, -0.1931;
     0, -0.0011, -0.1080, 0.0114, 0, 0;
     0, 0.0023, -0.3293, -0.226, 0, -0.0741;
     0, 0, 1, 0, 0, 0 ;
     0, 0, 0, 1, 0, 0;]; %状态空间方程线性化A矩阵系数
E=diag([1,1,1,1,1,1]);
u=(-(A+E)*U-pros/c);

== matlab function usv_sys/control rules ==
  data: k input; prox1_sign output; c input; e input; de input; sigma input
function prox1_sign= fcn(k, c,e,de,sigma)
s =c * e +de;
prox1_sign = (-1)* k * s - sigma * sign(s);

== matlab function usv_sys/USV_4dof_PID控制 ==
  data: eta input size=8*1; xdot output size=6*1; tau input; pos_dot output size=2*1
function [xdot,pos_dot] = usv(eta, tau)

% 线性化船舶模型
% Inputs:
% eta= [u v p r phi psi x y]'
% xdot= [du dv dp dr dphi dpsi]'
% pos_dot=[dx dy]'
% tau = [Xe Ye Ke Ne]' 
%

% where
% u     = surge velocity          (m/s)
% v     = sway velocity           (m/s)
% p     = roll velocity           (rad/s)
% r     = yaw velocity            (rad/s)
% phi   = roll angle              (rad)
% psi   = yaw angle               (rad)
%
% Xe is the surge external force (e.g. rudder and fin forces)
% Ye is the sway external force  
% Ke is the sway external force  
% Ne is the sway external force   

% Vessel Data
rho_water     =	1014.0;	        %	water density	[kg/m^3]	
rho_air		=	1.225	;	    %	air density		[kg/m^3]	
g				=	9.81;	        %	gravity constant	[m/s^2]	
deg2rad 		=	pi/180;	        %	degrees to radians	
rad2deg 		=	180/pi;	        %	rad to degrees		
ms2kt			=	3600/1852;	    % 	m/s to kt 			
kt2ms 		=	1852/3600;	    %	kt to m/s			
RPM2rads		=	2*pi/60;	    %	RPM to rad/s		
rads2RPM		=   60/(2*pi);	    %	rad/s to RPM		
HP2W			=	745.700;	    %	HP to Watt			


Lpp    =  51.5 ;                  % Length between perpendiculars垂直间长 [m]
B      =  8.6  ;                  % Beam over all 船宽 [m]
D	   =  2.3  ;                  % Draught吃水深度 [m]     

%Load condition (Modified by T.Perez)
disp   =  350.0;                   % Displacement 排水量 [m^3]
m      =  disp*rho_water;          % Mass [Kg]
Izz    =  47.934*10^6 ;            % Yaw Inertia偏航转动惯量
Ixx    =  2.3763*10^6 ;            % Roll Inertia横滚转动惯量
U_nom  =  8.0   ;	               % Speed nominal [m/sec]速度 (app 15kts) 
KM		=  4.47;	             %  [m] Transverse metacentre above keel 横倾复原力臂
KB		=  1.53;	             %  [m] Transverse centre of bouancy 浮心高度
gm 		=  1.1;	                 %  [m]	Transverse Metacenter 
bm 		=  KM - KB;
LCG       = 20.41 ;                % [m]	Longitudinal CG (from AP considered at the rudder stock)
VCG       = 3.36  ;                % [m]	Vertical  CG  above baseline
xG        = -3.38  ;               % coordinate of CG from the body fixed frame adopted for the PMM test  
zG  	    = -(VCG-D);          % coordinate of CG from the body fixed frame adopted for the PMM test  
m_xg	    = m * xG;
m_zg	    = m * zG;
Dp        = 1.6 ;                   % Propeller diameter [m]


% Data for surge equation 纵向（均为线性流体动力导数）
Xudot  	= -17400.0 ;  %-mx
Xuau     	= -1.96e+003 ;
Xvr    	=  0.33 * m ;
   
% Hydrodynamic coefficients in sway equation横向
Yvdot = -393000 ;  %-my
Ypdot = -296000 ; 
Yrdot = -1400000 ; %附加质量静距
Yauv  = -11800 ; 
Yur   =  131000 ; 
Yvav  = -3700 ; 
Yrar   =  0 ;
Yvar  = -794000 ; 
Yrav  = -182000 ; 
Ybauv =  10800 ; % Y_{\phi |v u|}
Ybaur =  251000 ; 
Ybuu  = -74 ; 


% Hydrodynamic coefficients in roll equation横摇水动力系数
Kvdot =  296000 ;
Kpdot = -774000 ;  %-Jxx
Krdot =  0 ;
Kauv  =  9260 ;
Kur   = -102000 ;
Kvav  =  29300 ;
Krar  =  0 ;
Kvar  =  621000 ;
Krav  =  142000 ;
Kbauv =  -8400 ;
Kbaur =  -196000 ;
Kbuu  =  -1180 ;
Kaup  =  -15500 ;
Kpap  =  -416000 ;
Kp    =  -500000 ;
Kb    =  0.776*m*g;
Kbbb  =  -0.325*m*g ;

% Hydrodynamic coefficients in yaw equation偏航水动力系数
Nvdot =  538000 ;   %-
Npdot =  0 ;
Nrdot = -38.7e6;    %jzz
Nauv  = -92000 ;
Naur  = -4710000 ;
Nvav  =  0 ;
Nrar  = -202000000 ;
Nvar  =  0 ;
Nrav  = -15600000 ;
Nbauv = -214000 ;
Nbuar = -4980000 ;
Nbuau = -8000 ;
%%%%%%%%%%%%%%%%%%%%%%%%%%%%%%%%%%%%%%%%%%%%%%%%%%%%%%%%%%%%%%%%%%%%%%%%%%%

% 定义输入
u   = eta(1);
v   = eta(2);
p  	= eta(3);   	
r  	= eta(4); 
b  	= eta(5); %phi roll 		
psi = eta(6);
x  	= eta(7);   	
y  	= eta(8); 
% 外部力与力矩
Xe  = tau(1);
Ye  = tau(2);
Ke  = tau(3);
Ne  = tau(4);

% Auxiliary variables辅助变量
au = abs(u);
av = abs(v); 
ar = abs(r); 
ap = abs(p); 
ab = abs(b);
L2 = Lpp^2; %参考面积？

% Total Mass Matrix 刚体质量矩阵
% x= [u v p r phi psi ]'
M =[ (m-Xudot)  0   0   0   0   0;
   0 (m-Yvdot) -(m*zG+Ypdot) (m*xG-Yrdot) 0 0;
   0 -(m*zG+Kvdot) (Ixx-Kpdot) -Krdot 0 0;
   0 (m*xG-Nvdot) -Npdot (Izz-Nrdot) 0 0;
   0 0 0 0 1 0; 
   0 0 0 0 0 1] ;
%转换矩阵
J=[cos(psi),-cos(b)*sin(psi);sin(psi),cos(b)*cos(psi)];
X=[u,v]';   
% Hydrodynamic forces without added mass terms(considered in the M matrix)
% 不考虑附加质量的水动力作用力 粘性流动动力（贵岛模型）
Xh  = Xuau*u*au+Xvr*v*r;

Yh = Yauv*au*v +  Yur*u*r + Yvav*v*av + Yvar*v*ar + Yrav*r*av + Ybauv*b*abs(u*v) + Ybaur*b*abs(u*r) + Ybuu*b*u^2;

Kh = Kauv*au*v +Kur*u*r + Kvav*v*av + Kvar*v*ar + Krav*r*av + Kbauv*b*abs(u*v) + Kbaur*b*abs(u*r) + Kbuu*b*u^2 +Kaup*au*p + Kpap*p*ap +Kp*p +Kbbb*b^3-(rho_water*g*gm*disp)*b;

Nh =Nauv*au*v + Naur*au*r +Nrar*r*ar + Nrav*r*av+Nbauv*b*abs(u*b) + Nbuar*b*u*ar + Nbuau*b*u*au;
 
% Rigid-body centripetal accelerations刚体运动产生的离心加速度影响
Xc =  m*(r*v+xG*r^2-zG*p*r);  
Yc = - m*u*r;
Kc =   m*zG*u*r;
Nc = - m*xG*u*r;

% Total forces
F1 = Xh+Xc+Xe;
F2 = Yh+Yc+Ye;
F4 = Kh+Kc+Ke;
F6 = Nh+Nc+Ne;

%运动学及动力学方程
pos_dot=J*X;
xdot = M\[F1; F2; F4; F6; p; r*cos(b)];

end

== matlab function usv_sys/actuaor1 ==
  data: v input; dphi input; angle input size=1*1; f output size=1*1
function f  = top(v, dphi, angle)

d=2;
f=1/2*v^2*1025*10*8.7*(angle+dphi*d/v);
end

== matlab function usv_sys/回转 ==
  data: v_x input; v_y input size=1*1; a_x input; a_y input; R output size=1*1
function R   = top(v_x, v_y,a_x,a_y)

R=sqrt((v_x^2+v_y^2)^3)/abs(v_x*a_y-v_y*a_x);
end
